simulink model "LCK_DanishV01"  (R2018b)
settings: Solver=FixedStepDiscrete  StartTime=0.0  StopTime=inf  FixedStep=0.01  RelTol=1e-3
PostLoadFcn:
  | if any(exist('dsrtsu_mdlpostloadfcn', 'file') ~= 0), dsrtsu_mdlpostloadfcn('Execute', bdroot); end
values from neighbouring files (symbols this model uses):
  C_DEG2RAD = 0.0175    [LCK_Macro.sldd]
  C_KPH2MPS = 0.2778    [LCK_Macro.sldd]
  C_NEARZERO = 0.0001    [LCK_Macro.sldd]
  C_ONE = 1.0    [LCK_Macro.sldd]
  C_RAD2DEG = 57.2958    [LCK_Macro.sldd]
  C_ZERO = 0.0    [LCK_Macro.sldd]
  k_accel_pedal_pos_per_speed_x : value not decoded    [LCK_LogicPara.sldd]
  k_accel_pedal_pos_per_speed_z : value not decoded    [LCK_LogicPara.sldd]
  k_brake_suprress_hold = 1000.0    [LCK_LogicPara.sldd]
  k_driver_appl_torque_filt = 50.0    [LCK_LogicPara.sldd]
  k_driver_suppression_hold_time = 3000.0    [LCK_LogicPara.sldd]
  k_hands_on_wheel_hold_msec = 500.0    [LCK_LogicPara.sldd]
  k_hands_on_wheel_torque_hi = 0.2    [LCK_LogicPara.sldd]
  k_hands_on_wheel_torque_lo = 0.15    [LCK_LogicPara.sldd]
  k_handsoff_delay_cycles = 50.0    [LCK_LogicPara.sldd]
  k_handsoff_torq_Lo_CR = 0.3    [LCK_LogicPara.sldd]
  k_handson_delay_cycles = 5.0    [LCK_LogicPara.sldd]
  k_HighAccel_suppress_hold = 3000.0    [LCK_LogicPara.sldd]
  k_HLR_suprress_hold = 3000.0    [LCK_LogicPara.sldd]
  k_hs_StrAng_CR_threshold_z : value not decoded    [LCK_LogicPara.sldd]
  k_LC_Exit_Switch = 0.0    [LCK_LogicPara.sldd]
  k_LCG_Configured = 1.0    [LCK_LogicPara.sldd]
  k_LCK_A0_Rdy2Act_UseConst = 0.0    [LCK_LogicPara.sldd]
  k_LCK_A0Fac_ActSta : value not decoded    [LCK_CtrlPara.sldd]
  k_LCK_A0Fac_DrvStm : value not decoded    [LCK_CtrlPara.sldd]
  k_LCK_A0Shift_LftCurv : value not decoded    [LCK_CtrlPara.sldd]
  k_LCK_A0Shift_RgtCurv : value not decoded    [LCK_CtrlPara.sldd]
  k_LCK_A0Shift_StraLan = 0.0    [LCK_CtrlPara.sldd]
  k_LCK_A0ShiftFac_Dy_LftCurv : value not decoded    [LCK_CtrlPara.sldd]
  k_LCK_A0ShiftFac_Dy_RgtCurv : value not decoded    [LCK_CtrlPara.sldd]
  k_LCK_A0ShiftFac_Vspd : value not decoded    [LCK_CtrlPara.sldd]
  k_LCK_accel_inhibit_thold = 35.0    [LCK_LogicPara.sldd]
  k_LCK_Active2Ready_Mask = 255.0    [LCK_LogicPara.sldd]
  k_LCK_CvatRateBks : value not decoded    [LCK_CtrlPara.sldd]
  k_LCK_CvatrBks : value not decoded    [LCK_CtrlPara.sldd]
  k_LCK_DFac_Dy : value not decoded    [LCK_CtrlPara.sldd]
  k_LCK_DFac_Dy_Curv : value not decoded    [LCK_CtrlPara.sldd]
  k_LCK_DFac_HaCurCen : value not decoded    [LCK_CtrlPara.sldd]
  k_LCK_DFac_HaCurSid : value not decoded    [LCK_CtrlPara.sldd]
  k_LCK_DFac_HadCurCen : value not decoded    [LCK_CtrlPara.sldd]
  k_LCK_DFac_HadCurSid : value not decoded    [LCK_CtrlPara.sldd]
  k_LCK_DFac_HadStrCen : value not decoded    [LCK_CtrlPara.sldd]
  k_LCK_DFac_HadStrSid : value not decoded    [LCK_CtrlPara.sldd]
  k_LCK_DFac_HaStrCen : value not decoded    [LCK_CtrlPara.sldd]
  k_LCK_DFac_HaStrSid : value not decoded    [LCK_CtrlPara.sldd]
  k_LCK_DFac_Rad : value not decoded    [LCK_CtrlPara.sldd]
  k_LCK_DFac_SA_CurCen : value not decoded    [LCK_CtrlPara.sldd]
  k_LCK_DFac_SA_CurSid : value not decoded    [LCK_CtrlPara.sldd]
  k_LCK_DFac_SA_StrCen : value not decoded    [LCK_CtrlPara.sldd]
  k_LCK_DFac_SA_StrSid : value not decoded    [LCK_CtrlPara.sldd]
  k_LCK_DFac_SS_CurCen : value not decoded    [LCK_CtrlPara.sldd]
  k_LCK_DFac_SS_CurSid : value not decoded    [LCK_CtrlPara.sldd]
  k_LCK_DFac_SS_StrCen : value not decoded    [LCK_CtrlPara.sldd]
  k_LCK_DFac_SS_StrSid : value not decoded    [LCK_CtrlPara.sldd]
  k_LCK_DFac_Vspd : value not decoded    [LCK_CtrlPara.sldd]
  k_LCK_DlyTm_DrvStim = 0.2    [LCK_CtrlPara.sldd]
  k_LCK_DTermMax = 2.0    [LCK_CtrlPara.sldd]
  k_LCK_DyBks_Curv : value not decoded    [LCK_CtrlPara.sldd]
  k_LCK_Enable_POOnly = 1.0    [LCK_LogicPara.sldd]
  k_LCK_Entry_DistBuffer = 0.1    [LCK_LogicPara.sldd]
  k_LCK_Fac_Vspd2RngThr_FalRec = 0.23    [LCK_CtrlPara.sldd]
  k_LCK_Ffw_CvatSwh = 0.0    [LCK_CtrlPara.sldd]
  k_LCK_Ffw_DyBks : value not decoded    [LCK_CtrlPara.sldd]
  k_LCK_Ffw_TimCon_CmdFlt = 0.0    [LCK_CtrlPara.sldd]
  k_LCK_FfwDeltaFac_Rad_Lft : value not decoded    [LCK_CtrlPara.sldd]
  k_LCK_FfwDeltaFac_Rad_Rgt : value not decoded    [LCK_CtrlPara.sldd]
  k_LCK_FfwDeltaFac_Vspd : value not decoded    [LCK_CtrlPara.sldd]
  k_LCK_FfwFac_CvatRate_Lft : value not decoded    [LCK_CtrlPara.sldd]
  k_LCK_FfwFac_CvatRate_Rgt : value not decoded    [LCK_CtrlPara.sldd]
  k_LCK_FfwFac_Dy : value not decoded    [LCK_CtrlPara.sldd]
  k_LCK_FfwFac_Rad_Lft : value not decoded    [LCK_CtrlPara.sldd]
  k_LCK_FfwFac_Rad_Rgt : value not decoded    [LCK_CtrlPara.sldd]
  k_LCK_FfwFac_Vspd : value not decoded    [LCK_CtrlPara.sldd]
  k_LCK_FfwTorq_Cvat : value not decoded    [LCK_CtrlPara.sldd]
  k_LCK_HAFac_ActSta : value not decoded    [LCK_CtrlPara.sldd]
  k_LCK_HAFac_DrvStm : value not decoded    [LCK_CtrlPara.sldd]
  k_LCK_HaloTime = 2000.0    [LCK_LogicPara.sldd]
  k_LCK_HaloTime_Switch = 0.0    [LCK_LogicPara.sldd]
  k_LCK_HARFac_ActSta : value not decoded    [LCK_CtrlPara.sldd]
  k_LCK_HARFac_DrvStm : value not decoded    [LCK_CtrlPara.sldd]
  k_LCK_Hed_DyBks : value not decoded    [LCK_CtrlPara.sldd]
  k_LCK_HedAngDiffX : value not decoded    [LCK_CtrlPara.sldd]
  k_LCK_HedAngRateDiffX : value not decoded    [LCK_CtrlPara.sldd]
  k_LCK_HndsOnWhel_DlyTm_Idl2Rdy = 0.0    [LCK_LogicPara.sldd]
  k_LCK_host_veh_width = 1.86    [LCK_LogicPara.sldd]
  k_LCK_Idle2Ready_Mask = 239.0    [LCK_LogicPara.sldd]
  k_LCK_Junc_SusTime = 1.0    [LCK_LogicPara.sldd]
  k_LCK_KpKdDecSlopeLmt = 10.0    [LCK_CtrlPara.sldd]
  k_LCK_KpKdIncSlopeLmt = 5.0    [LCK_CtrlPara.sldd]
  k_LCK_Lat_Ctrl_DFac_Lft = 1.0    [LCK_CtrlPara.sldd]
  k_LCK_Lat_Ctrl_DFac_Rgt = 1.05    [LCK_CtrlPara.sldd]
  k_LCK_Lat_Ctrl_Kd = 0.8    [LCK_CtrlPara.sldd]
  k_LCK_Lat_Ctrl_Ki = 0.5    [LCK_CtrlPara.sldd]
  k_LCK_Lat_Ctrl_Kp = 0.7    [LCK_CtrlPara.sldd]
  k_LCK_Lat_Ctrl_Kp_NearGain = 0.7    [LCK_CtrlPara.sldd]
  k_LCK_Lat_Ctrl_PFac_Lft = 1.0    [LCK_CtrlPara.sldd]
  k_LCK_Lat_Ctrl_PFac_Rgt = 1.05    [LCK_CtrlPara.sldd]
  k_LCK_Lat_Ctrl_TimCon_CmdFlt = 5.0    [LCK_CtrlPara.sldd]
  k_LCK_Lat_DFac_Rad : value not decoded    [LCK_CtrlPara.sldd]
  k_LCK_Lat_DFac_SS_Cur : value not decoded    [LCK_CtrlPara.sldd]
  k_LCK_Lat_DFac_SS_Str : value not decoded    [LCK_CtrlPara.sldd]
  k_LCK_Lat_DFac_Vspd : value not decoded    [LCK_CtrlPara.sldd]
  k_LCK_Lat_DyBks : value not decoded    [LCK_CtrlPara.sldd]
  k_LCK_Lat_IFac_Rad : value not decoded    [LCK_CtrlPara.sldd]
  k_LCK_Lat_IFac_Vspd : value not decoded    [LCK_CtrlPara.sldd]
  k_LCK_Lat_ILmtFac_Dy_CurvLan : value not decoded    [LCK_CtrlPara.sldd]
  k_LCK_Lat_ILmtFac_Dy_StraLan : value not decoded    [LCK_CtrlPara.sldd]
  k_LCK_Lat_ILmtFac_Rad : value not decoded    [LCK_CtrlPara.sldd]
  k_LCK_Lat_ILmtFac_Rad_NearGain = 1.0    [LCK_CtrlPara.sldd]
  k_LCK_Lat_ILmtFac_Vspd_CurvLan : value not decoded    [LCK_CtrlPara.sldd]
  k_LCK_Lat_ILmtFac_Vspd_StraLan : value not decoded    [LCK_CtrlPara.sldd]
  k_LCK_Lat_ITermLmt_Dy = 1.0    [LCK_CtrlPara.sldd]
  k_LCK_Lat_KpKdDecSlopeLmt = 10.0    [LCK_CtrlPara.sldd]
  k_LCK_Lat_KpKdIncSlopeLmt = 10.0    [LCK_CtrlPara.sldd]
  k_LCK_Lat_PFac_Dy_InnLftCur : value not decoded    [LCK_CtrlPara.sldd]
  k_LCK_Lat_PFac_Dy_InnRgtCur : value not decoded    [LCK_CtrlPara.sldd]
  k_LCK_Lat_PFac_Dy_OutLftCur : value not decoded    [LCK_CtrlPara.sldd]
  k_LCK_Lat_PFac_Dy_OutRgtCur : value not decoded    [LCK_CtrlPara.sldd]
  k_LCK_Lat_PFac_Dy_Str : value not decoded    [LCK_CtrlPara.sldd]
  k_LCK_Lat_PFac_Rad : value not decoded    [LCK_CtrlPara.sldd]
  ... (+153 more)
undefined symbols (not defined in the file or in its folder): k_LCK_CurvBks, K_LCK_SPA0A1A2_LMRngCmp_y
libraries: LateralControl_fcns_lib x58, simulink x24
(part 21 of 47)

== system LCK_DanishV01/Lateral_Control_Module/Adas_Lateral_Control_LCK_Core/Module 8/Module 0 ==
  Dy_1 : Inport
  Dy_0 : Inport  Port=2
  Lat_Rate : Inport  Port=3
  Vspd : Inport  Port=4
  Road_Radius : Inport  Port=5
  Steer_Spd : Inport  Port=6
  PosLan_Info : Inport  Port=7
  Bus Creator1 : BusCreator  Inputs=3
  Bus Creator2 : BusCreator  Inputs=3
  Bus Creator3 : BusCreator  Inputs=2
  Bus Creator4 : BusCreator  Inputs=3
  Bus Creator5 : BusCreator  Inputs=2
  Bus Creator6 : BusCreator  Inputs=2
  Bus Selector{1..3,5..7,17} (7 alike) : BusSelector  OutputSignals=signal1
  Bus Selector10 : BusSelector  OutputSignals=signal3
  Bus Selector11 : BusSelector  OutputSignals=signal3
  Bus Selector12 : BusSelector  OutputSignals=signal3
  Bus Selector{4,8..9,13} (4 alike) : BusSelector  OutputSignals=signal2
  Bus Selector14 : BusSelector  OutputSignals=Str_Flag,signal4,signal5,signal3
  D Gain : Subsystem
  "Definition  Fac 1 " : Subsystem
  Definition  Limit : Subsystem
  Definition Fac 2 : Subsystem
  Definition Fac 3 : Subsystem
  Definition Fac 4 : Subsystem
  Definition Fac 5 : Subsystem
  Definition Fac 6 : Subsystem
  I Gain : Subsystem
  Limitation of D Gain : Subsystem
  Limitation of P0 Gain : Subsystem
  Limitation of P1 Gain : Subsystem
  P0 Gain : Subsystem
  P1 Gain : Subsystem
  P_Gain : Outport
  I_Gain : Outport  Port=2
  D_Gain : Outport  Port=3
  ITerm_Limit : Outport  Port=4
  wires:
  Bus Selector14/4 -> Definition Fac 3/2(Inn_Cur_Flag_1)  "<signal3>"
  Dy_1/1 -> Definition Fac 3/3(Dy_1), "Definition  Fac 1 "/1(Dy_1)
  Dy_0/1 -> Definition  Limit/3(Dy_1), Definition Fac 2/1(Dy_0), "Definition  Fac 1 "/2(Dy_0)
  Lat_Rate/1 -> "Definition  Fac 1 "/3(Lat_Rate)
  PosLan_Info/1 -> Bus Selector14/1
  Vspd/1 -> Definition Fac 4/1(Vspd), Definition  Limit/2(Vspd)
  Road_Radius/1 -> Definition Fac 5/1(Road_Radius), Definition  Limit/1(Road_Radius)
  Steer_Spd/1 -> Definition Fac 6/1(Steer_Spd)
  Definition Fac 2/1(LatCtrl_P0Fac_Dy) -> P0 Gain/2(LatCtrl_P0Fac_Dy)
  P0 Gain/1(P0_Gain) -> Limitation of P0 Gain/1(P0_Gain)
  "Definition  Fac 1 "/1(LatCtrl_P0Fac_Asym) -> Bus Creator4/1
  "Definition  Fac 1 "/2(LatCtrl_P1Fac_Asym) -> Bus Creator4/2
  "Definition  Fac 1 "/3(LatCtrl_DFac_Asym) -> Bus Creator4/3
  Definition Fac 4/1(LatCtrl_PFac_Vspd) -> Bus Creator1/1
  Definition Fac 4/2(LatCtrl_IFac_Vspd) -> Bus Creator1/2
  Definition Fac 4/3(LatCtrl_DFac_Vspd) -> Bus Creator1/3
  Definition Fac 5/1(LatCtrl_PFac_Radius) -> Bus Creator2/1
  Definition Fac 5/2(LatCtrl_IFac_Radius) -> Bus Creator2/2
  Definition Fac 5/3(LatCtrl_DFac_Radius) -> Bus Creator2/3
  Definition Fac 6/1(LatCtrl_PFac_StrSpd) -> Bus Creator3/1
  Definition Fac 6/2(LatCtrl_DFac_StrSpd) -> Bus Creator3/2
  Definition  Limit/1(ITerm_Limit_1) -> Bus Creator5/1
  Definition  Limit/2(ITerm_Limit_0) -> Bus Creator5/2
  Bus Creator4/1 -> Bus Selector4/1, Bus Selector10/1, Bus Selector17/1
  Bus Selector17/1 -> P0 Gain/1(LatCtrl_P0Fac_Asym)  "<signal1>"
  Bus Creator1/1 -> Bus Selector1/1, Bus Selector5/1, Bus Selector8/1, Bus Selector11/1
  Bus Selector1/1 -> P0 Gain/3(LatCtrl_PFac_Vspd)  "<signal1>"
  Bus Selector2/1 -> P0 Gain/4(LatCtrl_PFac_Radius)  "<signal1>"
  Bus Creator2/1 -> Bus Selector12/1, Bus Selector6/1, Bus Selector2/1, Bus Selector9/1
  Bus Selector3/1 -> P0 Gain/5(LatCtrl_PFac_StrSpd)  "<signal1>"
  Bus Creator3/1 -> Bus Selector3/1, Bus Selector7/1, Bus Selector13/1
  P1 Gain/1(P1_Gain) -> Limitation of P1 Gain/1(P1_Gain)
  Limitation of P0 Gain/1(P0_Gain_Limited) -> Bus Creator6/1
  Limitation of P1 Gain/1(P1_Gain_Limited) -> Bus Creator6/2
  Bus Creator6/1 -> P_Gain/1
  Bus Selector4/1 -> P1 Gain/1(LatCtrl_P1Fac_Asym)  "<signal2>"
  Definition Fac 3/1(LatCtrl_P1Fac_Dy) -> P1 Gain/2(LatCtrl_P1Fac_Dy)
  Bus Selector5/1 -> P1 Gain/3(LatCtrl_PFac_Vspd)  "<signal1>"
  Bus Selector6/1 -> P1 Gain/4(LatCtrl_PFac_Radius)  "<signal1>"
  Bus Selector7/1 -> P1 Gain/5(LatCtrl_PFac_StrSpd)  "<signal1>"
  Bus Creator5/1 -> ITerm_Limit/1
  Bus Selector8/1 -> I Gain/1(LatCtrl_IFac_Vspd)  "<signal2>"
  Bus Selector9/1 -> I Gain/2(LatCtrl_IFac_Radius)  "<signal2>"
  Bus Selector10/1 -> D Gain/1(LatCtrl_DFac_Asym)  "<signal3>"
  Bus Selector11/1 -> D Gain/2(LatCtrl_DFac_Vspd)  "<signal3>"
  Bus Selector12/1 -> D Gain/3(LatCtrl_DFac_Radius)  "<signal3>"
  Bus Selector13/1 -> D Gain/4(LatCtrl_DFac_StrSpd)  "<signal2>"
  D Gain/1(D_Gain) -> Limitation of D Gain/1(D_Gain)
  Limitation of D Gain/1(D_Gain_Limited) -> D_Gain/1
  I Gain/1(I Gain) -> I_Gain/1
  Bus Selector14/2 -> Definition Fac 2/3(Inn_Cur_Flag_0)  "<signal4>"
  Bus Selector14/3 -> Definition Fac 3/1(Cur_Flag), Definition Fac 2/4(Cur_Flag)  "<signal5>"
  Bus Selector14/1 -> [Str_Flag], Definition Fac 2/2(Str_Flag)  "<Str_Flag>"
  [Str_Flag] -> Definition Fac 3/4(Str_Flag)
  [Str_Flag] -> Definition Fac 6/2(Str_Flag)
  [Str_Flag] -> Definition  Limit/4(Str_Flag)
